simulink model "Test"  (R2019b)
settings: Solver=ode45  StartTime=0.0  StopTime=10  RelTol=1e-3
values from neighbouring files (symbols this model uses):
  Kd1 = 20    [Fuzzy_Project.m]
  Kd2 = 15    [Fuzzy_Project.m]
  Kd3 = 15    [Fuzzy_Project.m]
  Ki1 = 0    [Fuzzy_Project.m]
  Ki2 = 30    [Fuzzy_Project.m]
  Ki3 = 30    [Fuzzy_Project.m]
  Kp1 = 30    [Fuzzy_Project.m]
  Kp2 = 40    [Fuzzy_Project.m]
  Kp3 = 50    [Fuzzy_Project.m]
  Pee_f = [-0.5 , -0.7 , 1.5]    [Fuzzy_Project.m]
  Pee_i = [0.5 , 0 , 1.5]    [Fuzzy_Project.m]
  T = 10    [Fuzzy_Project.m]
  t_b_q1 = 0.8    [Fuzzy_Project.m]
  t_b_q2 = 0.8    [Fuzzy_Project.m]
  t_b_q3 = 0.8    [Fuzzy_Project.m]
settings Model: Creator=Javad  LastModifiedBy=SARA
settings OptimizationCC: LifeSpan=inf
settings DebuggingCC: SFExecutionAtInitializationDiag=none  ArithmeticOperatorsInVariantConditions=warning
settings HardwareCC: ProdBitPerSizeT=32  ProdBitPerPtrDiffT=32  ProdWordSize=32  ProdHWDeviceType=Specified
settings SFSimCC: CustomCodeUndefinedFunction=UseInterfaceOnly
settings CodeAppCC: StateflowObjectComments=on

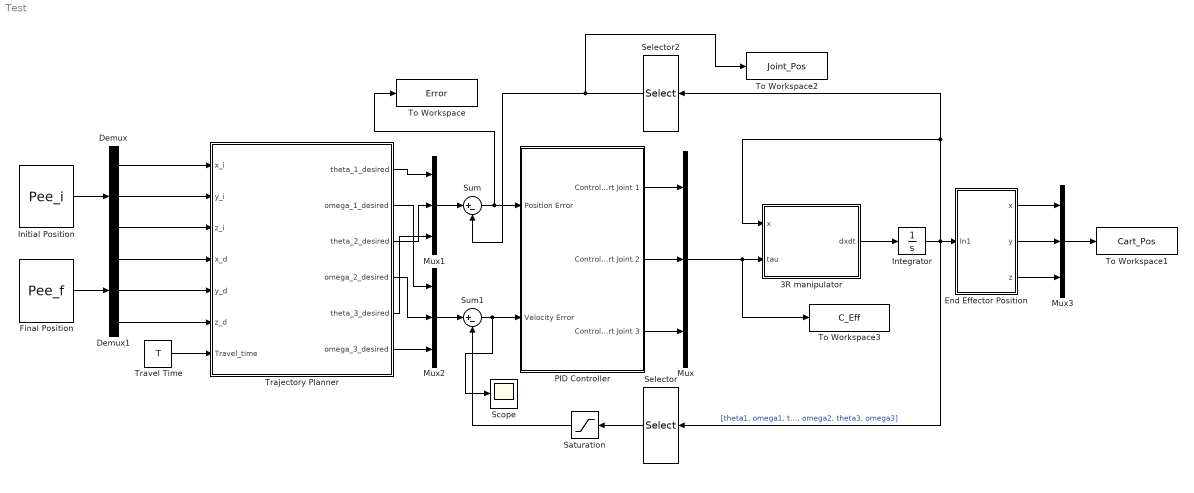
== system Test ==
  3R manipulator : MATLAB Function  TreatAsAtomicUnit=on
  Demux : Demux  Outputs=3
  Demux1 : Demux  Outputs=3
  End Effector Position : Subsystem
  Final Position : Constant  Value=Pee_f  VectorParams1D=off
  Initial Position : Constant  Value=Pee_i  VectorParams1D=off
  Integrator : Integrator  InitialCondition=[0;0;0.01;0;0;0]
  Mux{,1..3} (4 alike) : Mux  Inputs=3
  PID Controller : Subsystem
  Saturation : Saturate  UpperLimit=3  LowerLimit=-3
  Scope : Scope
  Selector : Selector  InputPortWidth=6  IndexOptions=Index vector (dialog)  Indices=[2 4 6]  OutputSizes=1
  Selector2 : Selector  InputPortWidth=6  IndexOptions=Index vector (dialog)  Indices=[1 3 5]  OutputSizes=1
  Sum : Sum  Inputs=|+-
  Sum1 : Sum  Inputs=|+-
  To Workspace : ToWorkspace  VariableName=Error  SaveFormat=Timeseries  SampleTime=-1
      settings: Save2DSignal=2-D array (concatenate along first dimension)
  To Workspace1 : ToWorkspace  VariableName=Cart_Pos  SaveFormat=Timeseries  SampleTime=-1
      settings: Save2DSignal=2-D array (concatenate along first dimension)
  To Workspace2 : ToWorkspace  VariableName=Joint_Pos  SaveFormat=Timeseries  SampleTime=-1
      settings: Save2DSignal=2-D array (concatenate along first dimension)
  To Workspace3 : ToWorkspace  VariableName=C_Eff  SaveFormat=Timeseries  SampleTime=-1
      settings: Save2DSignal=2-D array (concatenate along first dimension)
  Trajectory Planner : Subsystem
  "Travel Time " : Constant  Value=T
  wires:
  Initial Position/1 -> Demux/1
  Demux/1 -> Trajectory Planner/1(x_i)
  Demux/2 -> Trajectory Planner/2(y_i)
  Demux/3 -> Trajectory Planner/3(z_i)
  "Travel Time "/1 -> Trajectory Planner/7(Travel_time)
  Final Position/1 -> Demux1/1
  Demux1/1 -> Trajectory Planner/4(x_d)
  Demux1/2 -> Trajectory Planner/5(y_d)
  Demux1/3 -> Trajectory Planner/6(z_d)
  3R manipulator/1(dxdt) -> Integrator/1
  Integrator/1 -> End Effector Position/1(In1), Selector/1, Selector2/1, 3R manipulator/1(x)  "[theta1, omega1, theta2, omega2, theta3, omega3]"
  Mux/1 -> To Workspace3/1, 3R manipulator/2(tau)
  PID Controller/1(Control Effort Joint 1) -> Mux/1
  PID Controller/2(Control Effort Joint 2) -> Mux/2
  PID Controller/3(Control Effort Joint 3) -> Mux/3
  Trajectory Planner/1(theta_1_desired) -> Mux1/1
  Trajectory Planner/3(theta_2_desired) -> Mux1/2
  Trajectory Planner/5(theta_3_desired) -> Mux1/3
  Trajectory Planner/2(omega_1_desired) -> Mux2/1
  Trajectory Planner/4(omega_2_desired) -> Mux2/2
  Trajectory Planner/6(omega_3_desired) -> Mux2/3
  Sum/1 -> To Workspace/1, PID Controller/1(Position Error)
  Sum1/1 -> Scope/1, PID Controller/2(Velocity Error)
  Mux1/1 -> Sum/1
  Mux2/1 -> Sum1/1
  Selector/1 -> Saturation/1
  Selector2/1 -> To Workspace2/1, Sum/2
  Mux3/1 -> To Workspace1/1
  End Effector Position/1(x) -> Mux3/1
  End Effector Position/2(y) -> Mux3/2
  End Effector Position/3(z) -> Mux3/3
  Saturation/1 -> Sum1/2

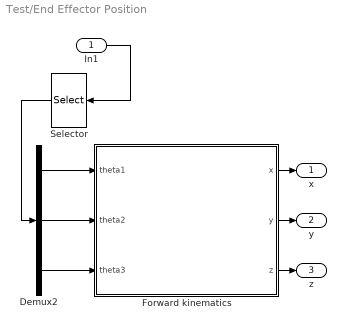
== system Test/End Effector Position ==
  In1 : Inport
  Demux2 : Demux  Outputs=3
  Forward kinematics : MATLAB Function  TreatAsAtomicUnit=on
  Selector : Selector  InputPortWidth=6  IndexOptions=Index vector (dialog)  Indices=[1 3 5]  OutputSizes=1
  x : Outport
  y : Outport  Port=2
  z : Outport  Port=3
  wires:
  Demux2/1 -> Forward kinematics/1(theta1)
  In1/1 -> Selector/1
  Forward kinematics/2(y) -> y/1
  Forward kinematics/3(z) -> z/1
  Forward kinematics/1(x) -> x/1
  Demux2/2 -> Forward kinematics/2(theta2)
  Demux2/3 -> Forward kinematics/3(theta3)
  Selector/1 -> Demux2/1

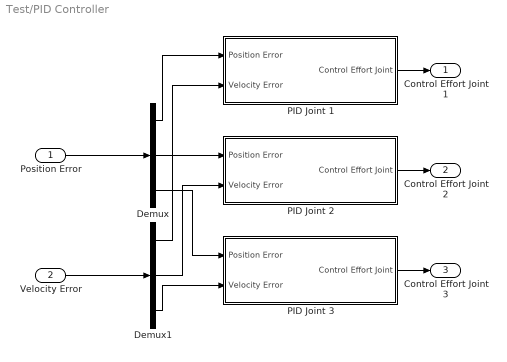
== system Test/PID Controller ==
  Position Error : Inport
  Velocity Error : Inport  Port=2
  Demux : Demux  Outputs=3
  Demux1 : Demux  Outputs=3
  PID Joint 1 : Subsystem
  PID Joint 2 : Subsystem
  PID Joint 3 : Subsystem
  Control Effort Joint 1 : Outport
  Control Effort Joint 2 : Outport  Port=2
  Control Effort Joint 3 : Outport  Port=3
  wires:
  PID Joint 2/1(Control Effort Joint) -> Control Effort Joint 2/1
  Demux1/3 -> PID Joint 3/2(Velocity Error)
  Demux/2 -> PID Joint 2/1(Position Error)
  Demux/3 -> PID Joint 3/1(Position Error)
  PID Joint 3/1(Control Effort Joint) -> Control Effort Joint 3/1
  Demux1/2 -> PID Joint 2/2(Velocity Error)
  Demux1/1 -> PID Joint 1/2(Velocity Error)
  Demux/1 -> PID Joint 1/1(Position Error)
  PID Joint 1/1(Control Effort Joint) -> Control Effort Joint 1/1
  Position Error/1 -> Demux/1
  Velocity Error/1 -> Demux1/1

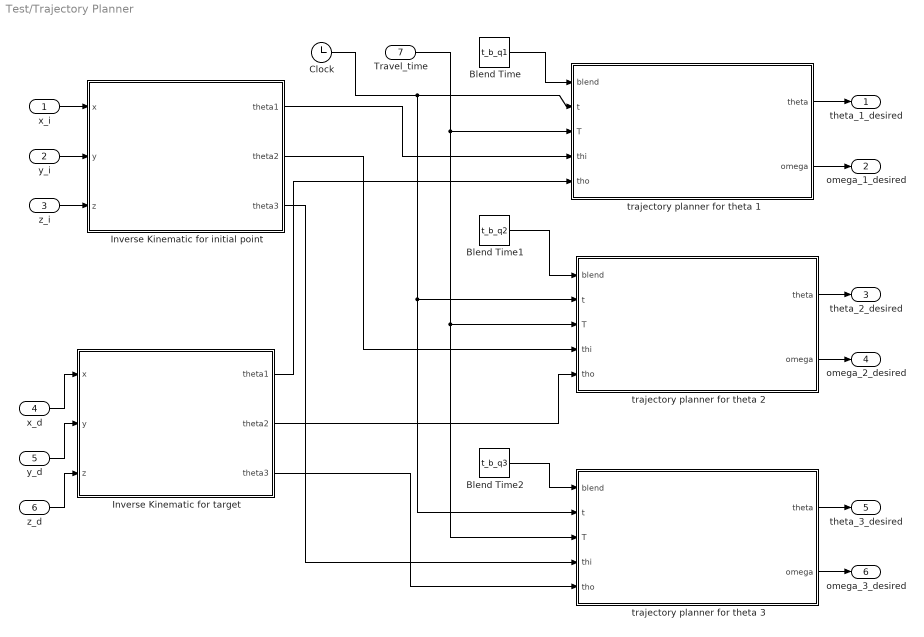
== system Test/Trajectory Planner ==
  x_i : Inport
  y_i : Inport  Port=2
  z_i : Inport  Port=3
  x_d : Inport  Port=4
  y_d : Inport  Port=5
  z_d : Inport  Port=6
  Travel_time : Inport  Port=7
  Blend Time : Constant  Value=t_b_q1
  Blend Time1 : Constant  Value=t_b_q2
  Blend Time2 : Constant  Value=t_b_q3
  Clock : Clock
  Inverse Kinematic for initial point : MATLAB Function  TreatAsAtomicUnit=on
  Inverse Kinematic for target : MATLAB Function  TreatAsAtomicUnit=on
  trajectory planner for theta 1 : MATLAB Function  TreatAsAtomicUnit=on
  trajectory planner for theta 2 : MATLAB Function  TreatAsAtomicUnit=on
  trajectory planner for theta 3 : MATLAB Function  TreatAsAtomicUnit=on
  theta_1_desired : Outport
  omega_1_desired : Outport  Port=2
  theta_2_desired : Outport  Port=3
  omega_2_desired : Outport  Port=4
  theta_3_desired : Outport  Port=5
  omega_3_desired : Outport  Port=6
  wires:
  trajectory planner for theta 1/2(omega) -> omega_1_desired/1
  y_i/1 -> Inverse Kinematic for initial point/2(y)
  trajectory planner for theta 1/1(theta) -> theta_1_desired/1
  Inverse Kinematic for initial point/1(theta1) -> trajectory planner for theta 1/4(thi)
  Inverse Kinematic for target/1(theta1) -> trajectory planner for theta 1/5(tho)
  x_i/1 -> Inverse Kinematic for initial point/1(x)
  z_i/1 -> Inverse Kinematic for initial point/3(z)
  Inverse Kinematic for initial point/2(theta2) -> trajectory planner for theta 2/4(thi)
  trajectory planner for theta 2/2(omega) -> omega_2_desired/1
  trajectory planner for theta 2/1(theta) -> theta_2_desired/1
  Inverse Kinematic for target/2(theta2) -> trajectory planner for theta 2/5(tho)
  Clock/1 -> trajectory planner for theta 1/2(t), trajectory planner for theta 3/2(t), trajectory planner for theta 2/2(t)
  Inverse Kinematic for target/3(theta3) -> trajectory planner for theta 3/5(tho)
  trajectory planner for theta 3/1(theta) -> theta_3_desired/1
  Inverse Kinematic for initial point/3(theta3) -> trajectory planner for theta 3/4(thi)
  Travel_time/1 -> trajectory planner for theta 1/3(T), trajectory planner for theta 2/3(T), trajectory planner for theta 3/3(T)
  trajectory planner for theta 3/2(omega) -> omega_3_desired/1
  Blend Time/1 -> trajectory planner for theta 1/1(blend)
  z_d/1 -> Inverse Kinematic for target/3(z)
  x_d/1 -> Inverse Kinematic for target/1(x)
  y_d/1 -> Inverse Kinematic for target/2(y)
  Blend Time1/1 -> trajectory planner for theta 2/1(blend)
  Blend Time2/1 -> trajectory planner for theta 3/1(blend)

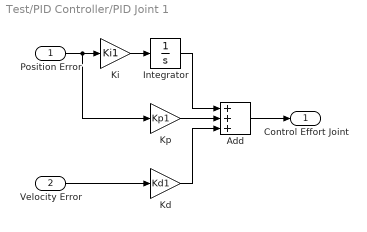
== system Test/PID Controller/PID Joint 1 ==
  Position Error : Inport
  Velocity Error : Inport  Port=2
  Add : Sum  Inputs=+++
  Integrator : Integrator
  Kd : Gain  Gain=Kd1
  Ki : Gain  Gain=Ki1
  Kp : Gain  Gain=Kp1
  Control Effort Joint : Outport
  wires:
  Kp/1 -> Add/2
  Add/1 -> Control Effort Joint/1
  Velocity Error/1 -> Kd/1
  Kd/1 -> Add/3
  Position Error/1 -> Ki/1, Kp/1
  Ki/1 -> Integrator/1
  Integrator/1 -> Add/1

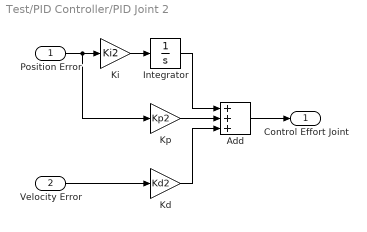
== system Test/PID Controller/PID Joint 2 ==
  Position Error : Inport
  Velocity Error : Inport  Port=2
  Add : Sum  Inputs=+++
  Integrator : Integrator
  Kd : Gain  Gain=Kd2
  Ki : Gain  Gain=Ki2
  Kp : Gain  Gain=Kp2
  Control Effort Joint : Outport
  wires:
  Kp/1 -> Add/2
  Add/1 -> Control Effort Joint/1
  Velocity Error/1 -> Kd/1
  Kd/1 -> Add/3
  Position Error/1 -> Ki/1, Kp/1
  Ki/1 -> Integrator/1
  Integrator/1 -> Add/1

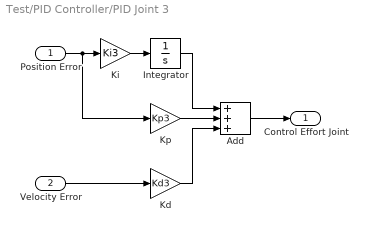
== system Test/PID Controller/PID Joint 3 ==
  Position Error : Inport
  Velocity Error : Inport  Port=2
  Add : Sum  Inputs=+++
  Integrator : Integrator
  Kd : Gain  Gain=Kd3
  Ki : Gain  Gain=Ki3
  Kp : Gain  Gain=Kp3
  Control Effort Joint : Outport
  wires:
  Kp/1 -> Add/2
  Add/1 -> Control Effort Joint/1
  Velocity Error/1 -> Kd/1
  Kd/1 -> Add/3
  Position Error/1 -> Ki/1, Kp/1
  Ki/1 -> Integrator/1
  Integrator/1 -> Add/1

== matlab function Test/Trajectory Planner/Inverse Kinematic for initial point ==
  data: x input; theta1 output; y input; z input; theta2 output; theta3 output
function [theta1, theta2, theta3] = inverse_kinematic(x, y, z)

L1=1.5; L2=0.8; L3=0.7;
theta1 = atan2(y, x);
theta3 = acos((x^2+y^2+(z-L1)^2-L2^2-L3^2)/(2*L2*L3));
phi = atan2(L3*sin(theta3), L3*cos(theta3)+L2);
disp(phi/pi*180)
theta2 = asin((z-L1)*cos(phi)/(L3*cos(theta3)+L2))-phi;

end

== matlab function Test/3R manipulator ==
  data: x input size=[6,1]; dxdt output size=[6,1]; tau input size=[3,1]

function dxdt = Plant_3R (x, tau)
th1 = x(1);
th1_d = x(2);
th2 = x(3);
th2_d = x(4);
th3 = x(5);
th3_d = x(6);
dxdt = zeros(6,1);
dxdt(1) = th1_d;
dxdt(2) = (2.4e+3*tau(1)-670.0*th1_d*th2_d*sin(th3)+...
    290.0*th1_d*th2_d*sin(2.0*th2+2.0*th3)+...
    290.0*th1_d*th3_d*sin(2.0*th2+2.0*th3)+...
    670.0*th1_d*th2_d*sin(2.0*th2+th3)+...
    380.0*th1_d*th2_d*sin(2.0*th2))/(340.0*cos(2.0*th2+th3)+...
    190.0*cos(2.0*th2)+340.0*cos(th3)+150.0*cos(2.0*th2+2.0*th3)+1.5e+3);
dxdt(3) = th2_d;
dxdt(4) = -0.38*sin(2.0*th2)*th1_d^2-18.0*cos(th2)+4.7*tau(2)-4.7*tau(3);
dxdt(5) = th3_d;
dxdt(6) = 16.0*cos(th2-1.0*th3)+85.0*cos(th2+th3)+18.0*cos(th2)-...
    0.86*th1_d^2*sin(th3)-1.7*th2_d^2*sin(th3)+...
    0.32*th1_d^2*sin(2.0*th2-1.0*th3)-...
    0.38*th1_d^2*sin(2.0*th2+2.0*th3)-...
    0.54*th1_d^2*sin(2.0*th2+th3)+0.38*th1_d^2*sin(2.0*th2)+...
    11.0*tau(3)-4.7*tau(2);

end

== matlab function Test/Trajectory Planner/trajectory planner for theta 1 ==
  data: blend input; t input; theta output; T input; thi input; tho input; omega output
function [theta, omega] = trajectory_planner(blend, t, T, thi, tho)
%t is the current time
%T is the toal time of the movement. 
%thi is the initial angle
%tho is the target angle
% blend = 1;

V_max = (tho-thi)/(T-blend);
a = V_max/blend;

if t<=blend
    alpha = a;
    omega = a*t;
    theta = 1/2*a*t.^2+thi;
elseif t<=(T-blend)
    alpha = 0;
    omega = V_max;
    theta = 1/2*a*blend^2+thi+V_max.*(t-blend);
else
    alpha = -a;
    omega = V_max-a.*(t-(T-blend));
    theta = -1/2*a.*(t-(T-blend)).^2+V_max*(t-(T-blend))+1/2*a*blend^2+thi+...
        V_max*(T-2*blend);
end
    
end

== matlab function Test/Trajectory Planner/trajectory planner for theta 2 ==
  data: blend input; t input; theta output; T input; thi input; tho input; omega output
function [theta, omega] = trajectory_planner(blend, t, T, thi, tho)
%t is the current time
%T is the toal time of the movement. 
%thi is the initial angle
%tho is the target angle
blend = 1;

V_max = (tho-thi)/(T-blend);
a = V_max/blend;

if t<=blend
    alpha = a;
    omega = a*t;
    theta = 1/2*a*t.^2+thi;
elseif t<=(T-blend)
    alpha = 0;
    omega = V_max;
    theta = 1/2*a*blend^2+thi+V_max.*(t-blend);
else
    alpha = -a;
    omega = V_max-a.*(t-(T-blend));
    theta = -1/2*a.*(t-(T-blend)).^2+V_max*(t-(T-blend))+1/2*a*blend^2+thi+...
        V_max*(T-2*blend);
end
    
end

== matlab function Test/Trajectory Planner/trajectory planner for theta 3 ==
  data: blend input; t input; theta output; T input; thi input; tho input; omega output
function [theta, omega] = trajectory_planner(blend, t, T, thi, tho)
%t is the current time
%T is the toal time of the movement. 
%thi is the initial angle
%tho is the target angle
blend = 1;

V_max = (tho-thi)/(T-blend);
a = V_max/blend;

if t<=blend
    alpha = a;
    omega = a*t;
    theta = 1/2*a*t.^2+thi;
elseif t<=(T-blend)
    alpha = 0;
    omega = V_max;
    theta = 1/2*a*blend^2+thi+V_max.*(t-blend);
else
    alpha = -a;
    omega = V_max-a.*(t-(T-blend));
    theta = -1/2*a.*(t-(T-blend)).^2+V_max*(t-(T-blend))+1/2*a*blend^2+thi+...
        V_max*(T-2*blend);
end
    
end

== matlab function Test/Trajectory Planner/Inverse Kinematic for target ==
  data: x input; theta1 output; y input; z input; theta2 output; theta3 output
function [theta1, theta2, theta3] = inverse_kinematic(x, y, z)

L1=1.5; L2=0.8; L3=0.7;
theta1 = atan2(y, x);
theta3 = acos((x^2+y^2+(z-L1)^2-L2^2-L3^2)/(2*L2*L3));
phi = atan2(L3*sin(theta3), L3*cos(theta3)+L2);
disp(phi/pi*180)
theta2 = asin((z-L1)*cos(phi)/(L3*cos(theta3)+L2))-phi;

end

== matlab function Test/End Effector Position/Forward kinematics ==
  data: x output; theta1 input; y output; theta2 input; theta3 input; z output
function [x, y, z] = fcn(theta1, theta2, theta3)
L1=1.5; L2=0.8; L3=0.7;T_01 = [cos(theta1) -sin(theta1) 0  0;
        sin(theta1)  cos(theta1) 0  0;
        0            0           1  0;
        0            0           0  1];
    
T_12 = [cos(theta2) -sin(theta2) 0  0;
        0            0          -1  0;
        sin(theta2)  cos(theta2) 0  0;
        0            0           0  1];
    
T_23 = [cos(theta3) -sin(theta3) 0  L2;
        sin(theta3)  cos(theta3) 0  0;
        0            0           1  0;
        0            0           0  1];

T_34 = [1            0           0  L3;
        0            1           0  0;
        0            0           1  0;
        0            0           0  1];
    
T_04 = (T_01*T_12*T_23*T_34);

x = T_04(1,4);
y = T_04(2,4);
z = T_04(3,4)+L1;
end
